simulink model "acDynModelGolfTenueModale2"  (R2019a)
settings: Solver=VariableStepAuto  StartTime=0.0  StopTime=10  RelTol=1e-3
values from neighbouring files (symbols this model uses):
  A6 = Acm(iVa:end, iVa:end)    [mainProjetCADV_2a.m]
  alphaTrim = trimVal(2)    [mainProjetCADV_2a.m]
  B6 = Bcm(iVa:end)    [mainProjetCADV_2a.m]
  Cobs = [C6(1,:); C6(3,:); C6(4,:)]    [mainProjetCADV_2a.m]
  dPHRTrim = trimVal(1)    [mainProjetCADV_2a.m]
  dthrIdle = 0.1    [mainProjetCADV_2a.m]
  hTrim = hTrimFL*FL2M    [mainProjetCADV_2a.m]
  K6 = place(A6,B6,[dp, conj(dp), -3.3965 + 0.1541i, -3.3965 - 0.1541i, -5, -6])    [mainProjetCADV_2a.m]
  K_i = K_aug(end)    [mainProjetCADV_2a.m]
  K_x = K_aug(1:end-1)    [mainProjetCADV_2a.m]
  km = trim.kmass(choix)    [utGetTrimPoint.m]
  KTS2MS = 1852 / 3600    (= 0.514444444444)    [mainProjetCADV_2a.m]    (also in utAcDynamicsFunction.m)
  L6 = L6t'    [mainProjetCADV_2a.m]
  ms = trim.mStat(choix)    [utGetTrimPoint.m]
  RAD2DEG = 180/pi    (= 57.2957795131)    [mainProjetCADV_2a.m]    (also in utAcDynamicsFunction.m)
  thetaTrim = trimVal(3)    [mainProjetCADV_2a.m]
  uTrim = zeros(TOTAL_CMD, 1)    [mainProjetCADV_2a.m]
  VaTrim = utEas2Tas(Eas_KTS*KTS2MS, hTrimFL*FL2M)    [mainProjetCADV_2a.m]
  xTrim = zeros(TOTAL_SV, 1)    [mainProjetCADV_2a.m]
undefined symbols (not defined in the file or in its folder): aircraftChosen, Eas_KTS, Kd, Ki, Kp
settings Model: Creator=bourdiul  LastModifiedBy=ulyss

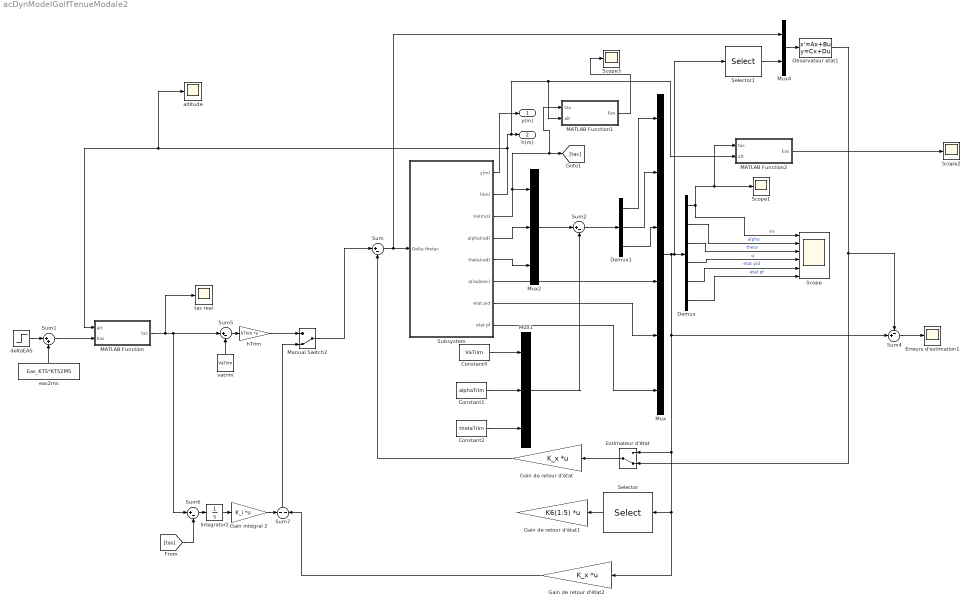
== system acDynModelGolfTenueModale2 ==
  Constant1 : Constant  Value=alphaTrim
  Constant2 : Constant  Value=thetaTrim
  Constant4 : Constant  Value=VaTrim
  Demux : Demux  Outputs=6
  Demux1 : Demux  Outputs=3
  Erreurs d'estimation1 : Scope
  Estimateur d'état : ManualSwitch  CurrentSetting=0
  Gain de retour d'état : Gain  Gain=K_x  Multiplication=Matrix(K*u) (u vector)
  Gain de retour d'état1 : Gain  Gain=K6(1:5)  Multiplication=Matrix(K*u) (u vector)
  Gain de retour d'état2 : Gain  Gain=K_x  Multiplication=Matrix(K*u) (u vector)
  Gain intégral 2 : Gain  Gain=K_i  Multiplication=Matrix(K*u) (u vector)
  Integrator2 : Integrator
  MATLAB Function : MATLAB Function  TreatAsAtomicUnit=on
  MATLAB Function1 : MATLAB Function  TreatAsAtomicUnit=on
  MATLAB Function2 : MATLAB Function  TreatAsAtomicUnit=on
  Manual Switch2 : ManualSwitch  CurrentSetting=0
  Mux : Mux  Inputs=6
  Mux1 : Mux  Inputs=3
  Mux2 : Mux  Inputs=3
  Mux4 : Mux  Inputs=2
  Observateur etat1 : StateSpace  A=A6-L6*Cobs  B=[B6, L6]  C=eye(6)  D=zeros(6,4)  InitialCondition=0
  Scope : Scope  NumInputPorts=6
  Scope1 : Scope
  Scope2 : Scope
  Scope3 : Scope
  Selector : Selector  InputPortWidth=6  IndexOptions=Index vector (dialog)  Indices=[1:5]  OutputSizes=1
  Selector1 : Selector  InputPortWidth=6  IndexOptions=Index vector (dialog)  Indices=[1,3,4]  OutputSizes=1
  Subsystem : Subsystem
  Sum{,2,5..6} (4 alike) : Sum  Inputs=|+-
  Sum1 : Sum  Inputs=|++
  Sum4 : Sum  Inputs=-+|
  Sum7 : Sum  Inputs=-|-
  altitude : Scope
  deltaEAS : Step  Time=0  After=5  SampleTime=0
  eas2ms : Constant  Value=Eas_KTS*KTS2MS
  hTrim : Gain  Gain=hTrim  Multiplication=Matrix(K*u) (u vector)
  tas real : Scope
  vatrim : Constant  Value=VaTrim
  y(m) : Outport
  h(m) : Outport  Port=2
  wires:
  Sum/1 -> Mux4/1, Subsystem/1("Delta thetac ")
  Demux/6 -> Scope/6  "etat pf"
  Demux/1 -> Scope/1, MATLAB Function2/1(tas), Scope1/1  "Va"
  Observateur etat1/1 -> Sum4/1, Estimateur d'état/2
  Mux/1 -> Selector1/1, Demux/1, Estimateur d'état/1, Gain de retour d'état2/1, Selector/1, Sum4/2
  Demux/2 -> Scope/2  "alpha"
  Sum2/1 -> Demux1/1
  Demux/4 -> Scope/4  "q"
  Estimateur d'état/1 -> Gain de retour d'état/1
  Constant1/1 -> Mux1/2
  Gain de retour d'état/1 -> Sum/2
  Subsystem/3(Va(m/s)) -> MATLAB Function1/1(tas), [tas], Mux2/1
  Sum4/1 -> Erreurs d'estimation1/1
  Demux1/3 -> Mux/3
  Subsystem/4(alpha(rad)) -> Mux2/2
  Subsystem/7(etat pid) -> Mux/5
  Constant4/1 -> Mux1/1
  Subsystem/8("etat pf ") -> Mux/6
  Demux/3 -> Scope/3  "theta"
  Demux/5 -> Scope/5  "etat pid"
  Mux1/1 -> Sum2/2
  Subsystem/2(h(m)) -> MATLAB Function1/2(alt), MATLAB Function2/2(alt), h(m)/1, altitude/1, MATLAB Function/1(alt)
  Constant2/1 -> Mux1/3
  Demux1/1 -> Mux/1
  Subsystem/5(theta(rad)) -> Mux2/3
  Subsystem/1(y(m)) -> y(m)/1
  Demux1/2 -> Mux/2
  Subsystem/6(q(rad/sec)) -> Mux/4
  Mux2/1 -> Sum2/1
  Sum7/1 -> Manual Switch2/2
  Integrator2/1 -> Gain intégral 2/1
  Sum1/1 -> MATLAB Function/2(Eas)
  Gain intégral 2/1 -> Sum7/1
  deltaEAS/1 -> Sum1/1
  MATLAB Function/1(tas) -> tas real/1, Sum5/1, Sum6/1
  vatrim/1 -> Sum5/2
  eas2ms/1 -> Sum1/2
  [tas] -> Sum6/2
  Sum5/1 -> hTrim/1
  Sum6/1 -> Integrator2/1
  hTrim/1 -> Manual Switch2/1
  Manual Switch2/1 -> Sum/1
  Selector/1 -> Gain de retour d'état1/1
  Selector1/1 -> Mux4/2
  Mux4/1 -> Observateur etat1/1
  Gain de retour d'état2/1 -> Sum7/2
  MATLAB Function2/1(Eas) -> Scope2/1
  MATLAB Function1/1(Eas) -> Scope3/1

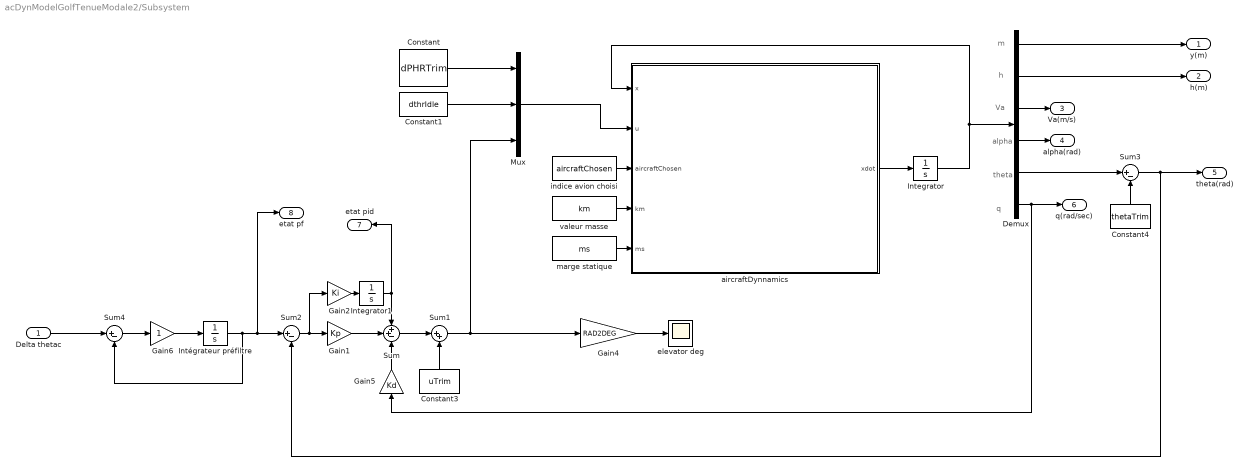
== system acDynModelGolfTenueModale2/Subsystem ==
  note: m
  note: h
  note: Va
  note: alpha
  note: theta
  note: q
  "Delta thetac " : Inport
  Constant : Constant  Value=dPHRTrim
  Constant1 : Constant  Value=dthrIdle
  Constant3 : Constant  Value=uTrim
  Constant4 : Constant  Value=thetaTrim
  Demux : Demux  Outputs=6
  Gain1 : Gain  Gain=Kp
  Gain2 : Gain  Gain=Ki
  Gain4 : Gain  Gain=RAD2DEG
  Gain5 : Gain  Gain=Kd
  Gain6 : Gain
  Integrator : Integrator  InitialCondition=xTrim
  Integrator1 : Integrator
  Intégrateur préfiltre : Integrator
  Mux : Mux  Inputs=3
  Sum : Sum  Inputs=++-
  Sum1 : Sum  Inputs=|++
  Sum2 : Sum  Inputs=|+-
  Sum3 : Sum  Inputs=|+-
  Sum4 : Sum  Inputs=|+-
  aircraftDynnamics : MATLAB Function  TreatAsAtomicUnit=on
  elevator deg : Scope
  indice avion choisi : Constant  Value=aircraftChosen
  marge statique : Constant  Value=ms
  valeur masse : Constant  Value=km
  y(m) : Outport
  h(m) : Outport  Port=2
  Va(m/s) : Outport  Port=3
  alpha(rad) : Outport  Port=4
  theta(rad) : Outport  Port=5
  q(rad/sec) : Outport  Port=6
  etat pid : Outport  Port=7
  "etat pf " : Outport  Port=8
  wires:
  aircraftDynnamics/1(xdot) -> Integrator/1
  "Delta thetac "/1 -> Sum4/1
  Sum/1 -> Sum1/1
  Sum1/1 -> Mux/3, Gain4/1
  Sum4/1 -> Gain6/1
  Gain2/1 -> Integrator1/1
  Constant/1 -> Mux/1
  Integrator1/1 -> etat pid/1, Sum/1
  Integrator/1 -> aircraftDynnamics/1(x), Demux/1
  Demux/6 -> q(rad/sec)/1, Gain5/1
  Demux/1 -> y(m)/1
  Sum2/1 -> Gain2/1, Gain1/1
  Mux/1 -> aircraftDynnamics/2(u)
  indice avion choisi/1 -> aircraftDynnamics/3(aircraftChosen)
  Demux/3 -> Va(m/s)/1
  Gain4/1 -> elevator deg/1
  marge statique/1 -> aircraftDynnamics/5(ms)
  Gain5/1 -> Sum/3
  valeur masse/1 -> aircraftDynnamics/4(km)
  Gain1/1 -> Sum/2
  Demux/4 -> alpha(rad)/1
  Constant3/1 -> Sum1/2
  Gain6/1 -> Intégrateur préfiltre/1
  Demux/2 -> h(m)/1
  Intégrateur préfiltre/1 -> "etat pf "/1, Sum2/1, Sum4/2
  Demux/5 -> Sum3/1
  Constant4/1 -> Sum3/2
  Constant1/1 -> Mux/2
  Sum3/1 -> theta(rad)/1, Sum2/2

== matlab function acDynModelGolfTenueModale2/MATLAB Function ==
  data: alt input; Eas input; tas output
function tas = utEas2tas(alt, Eas)
    %tas, Eas (%equivalent vitesse) en m/s
    %alt en m
    %cf. http://www.hochwarth.com/misc/AviationCalculator.html
    tas = sqrt(utRho(0)/utRho(alt))*Eas;
end

== matlab function acDynModelGolfTenueModale2/Subsystem/aircraftDynnamics ==
  data: x input; u input; xdot output; aircraftChosen input; km input; ms input
function xdot = aircraftDynamics(x,u, aircraftChosen,km,ms)
    TOTAL_SV = 6;
    xIn = zeros(TOTAL_SV,1);
    xIn = x;
    
	TOTAL_CMD = 3;
    uIn = zeros(TOTAL_CMD,1);
    uIn = u;
    
    xdot = utAcDynamicsFunction(xIn,uIn, aircraftChosen,km,ms);
end %aircraftDynamics

== matlab function acDynModelGolfTenueModale2/MATLAB Function1 ==
  data: tas input; alt input; Eas output
function Eas = utTas2Eas(tas, alt)
    %tas, Eas(%equivalent vitesse) en m/s
    %alt en m
    %cf. http://www.hochwarth.com/misc/AviationCalculator.html
    Eas = sqrt(utRho(alt)/utRho(0))*tas;
end

== matlab function acDynModelGolfTenueModale2/MATLAB Function2 ==
  data: tas input; alt input; Eas output
function Eas = utTas2Eas(tas, alt)
    %tas, Eas(%equivalent vitesse) en m/s
    %alt en m
    %cf. http://www.hochwarth.com/misc/AviationCalculator.html
    Eas = sqrt(utRho(alt)/utRho(0))*tas;
end
